simulink model "SimulationBangBangModel"  (R2024a)
settings: Solver=FixedStepAuto  StartTime=0.0  StopTime=tFinal_s  FixedStep=deltaT_s  RelTol=1e-3
values from neighbouring files (symbols this model uses):
  K = 49    [Step01_SimulationBangBangSetupModel.m]    (also in Step02a_SimulationBangBangHysteresisSetupModel.m)
  Tambient_C = 24.1875    [Step01_SimulationBangBangSetupModel.m]    (also in Step02a_SimulationBangBangHysteresisSetupModel.m)
  u_ON = 1    [Step01_SimulationBangBangSetupModel.m]    (also in Step02a_SimulationBangBangHysteresisSetupModel.m)
libraries: TemperatureControlLibrary x2
settings Model: Creator=chris  LastModifiedBy=chris

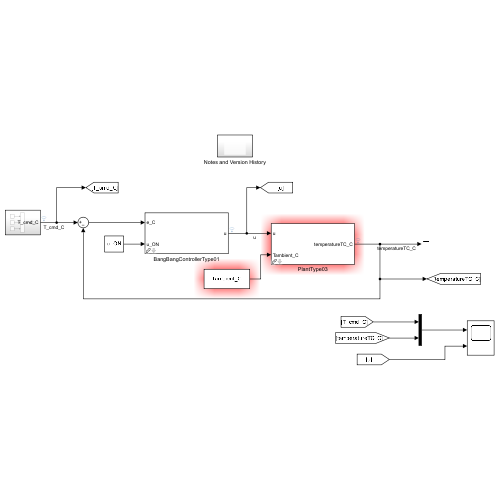
[thumbnail: Simulink's stored preview of the top-level diagram]
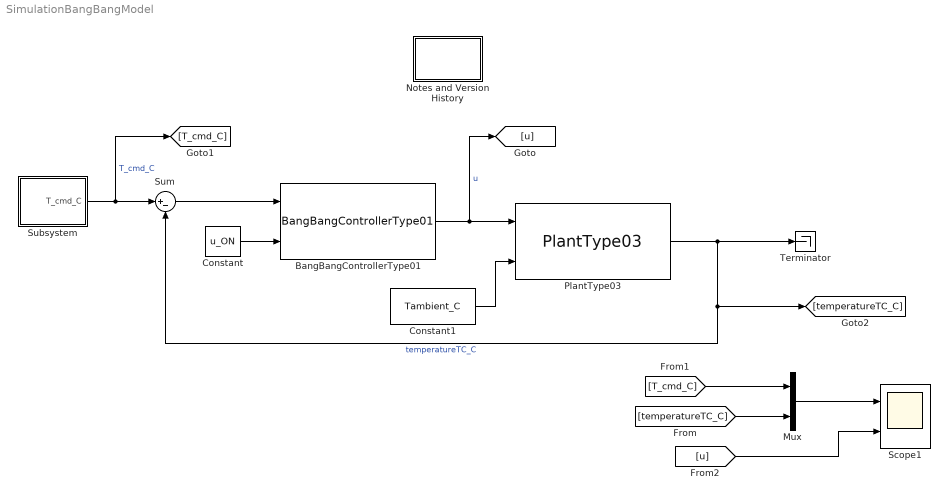
== system SimulationBangBangModel ==
  BangBangControllerType01 : TemperatureControlLibrary/BangBangControllerType01
  Constant : Constant  Value=u_ON
  Constant1 : Constant  Value=Tambient_C
  Mux : Mux  Inputs=2
  Notes and Version History : Subsystem
  PlantType03 : TemperatureControlLibrary/PlantType03  wn=wn  zeta=zeta  K=K  Tdelay_s=Tdelay_s
  Scope1 : Scope  NumInputPorts=2
  Subsystem : Subsystem
  Sum : Sum  Inputs=|+-
  Terminator : Terminator
  wires:
  BangBangControllerType01/1 -> [u], PlantType03/1  "u"
  PlantType03/1 -> Terminator/1, [temperatureTC_C], Sum/2  "temperatureTC_C"
  Sum/1 -> BangBangControllerType01/1
  Constant/1 -> BangBangControllerType01/2
  Subsystem/1(T_cmd_C) -> [T_cmd_C], Sum/1  "T_cmd_C"
  Mux/1 -> Scope1/1
  [temperatureTC_C] -> Mux/2
  [T_cmd_C] -> Mux/1
  [u] -> Scope1/2
  Constant1/1 -> PlantType03/2

== system SimulationBangBangModel/Notes and Version History ==
  note: Christopher Lum
      | lum@uw.edu
      |
      | Version History
      | 01/23/25: Created

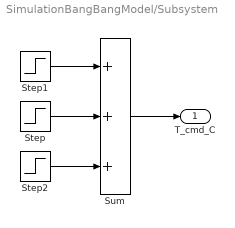
== system SimulationBangBangModel/Subsystem ==
  Step : Step  Time=2.5*60  After=-5  SampleTime=0
  Step1 : Step  Time=5  After=45  SampleTime=0
  Step2 : Step  Time=250  After=10  SampleTime=0
  Sum : Sum  Inputs=+++
  T_cmd_C : Outport
  wires:
  Step2/1 -> Sum/3
  Sum/1 -> T_cmd_C/1
  Step/1 -> Sum/2
  Step1/1 -> Sum/1
